simulink model "Check2_3"  (R2016b)
settings: Solver=VariableStepAuto  StartTime=0.0  StopTime=2  RelTol=1e-3
values from neighbouring files (symbols this model uses):
  h = 0.005    [Lab2.m]
  K = (K1 + K2) / 2    (= 15.4249961351)    [Lab2.m]
  kz1 = 15.2    [Lab2.m]
  kz2 = 4.22    [Lab2.m]
  kz3 = 1.73    [Lab2.m]
  tau = sqrt(tau1*tau2)    [Lab2.m]
  z1 = int(min_index)    [Lab2.m]
  z2 = z1 / 2    [Lab2.m]
  z3 = z1 / 3    [Lab2.m]
settings Model: Creator=EE103  LastModifiedBy=EE103

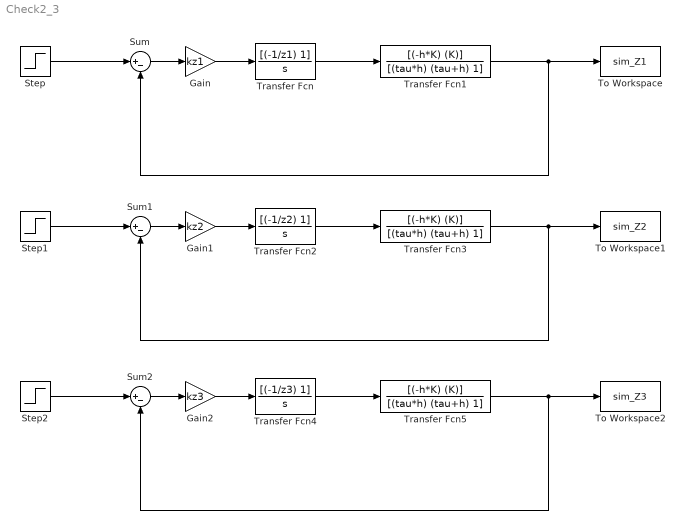
== system Check2_3 ==
  Gain : Gain  Gain=kz1
  Gain1 : Gain  Gain=kz2
  Gain2 : Gain  Gain=kz3
  Step : Step  Time=0  After=50  SampleTime=0.01
  Step1 : Step  Time=0  After=50  SampleTime=0.01
  Step2 : Step  Time=0  After=50  SampleTime=0.01
  Sum : Sum  Inputs=|+-
  Sum1 : Sum  Inputs=|+-
  Sum2 : Sum  Inputs=|+-
  To Workspace : ToWorkspace  VariableName=sim_Z1  SaveFormat=Timeseries  SampleTime=-1
  To Workspace1 : ToWorkspace  VariableName=sim_Z2  SaveFormat=Timeseries  SampleTime=-1
  To Workspace2 : ToWorkspace  VariableName=sim_Z3  SaveFormat=Timeseries  SampleTime=-1
  Transfer Fcn : TransferFcn  Numerator=[(-1/z1) 1]  Denominator=[1 0]
  Transfer Fcn1 : TransferFcn  Numerator=[(-h*K) (K)]  Denominator=[(tau*h) (tau+h) 1]
  Transfer Fcn2 : TransferFcn  Numerator=[(-1/z2) 1]  Denominator=[1 0]
  Transfer Fcn3 : TransferFcn  Numerator=[(-h*K) (K)]  Denominator=[(tau*h) (tau+h) 1]
  Transfer Fcn4 : TransferFcn  Numerator=[(-1/z3) 1]  Denominator=[1 0]
  Transfer Fcn5 : TransferFcn  Numerator=[(-h*K) (K)]  Denominator=[(tau*h) (tau+h) 1]
  wires:
  Step/1 -> Sum/1
  Sum/1 -> Gain/1
  Transfer Fcn/1 -> Transfer Fcn1/1
  Transfer Fcn1/1 -> Sum/2, To Workspace/1
  Step1/1 -> Sum1/1
  Sum1/1 -> Gain1/1
  Transfer Fcn2/1 -> Transfer Fcn3/1
  Transfer Fcn3/1 -> Sum1/2, To Workspace1/1
  Step2/1 -> Sum2/1
  Sum2/1 -> Gain2/1
  Transfer Fcn4/1 -> Transfer Fcn5/1
  Transfer Fcn5/1 -> Sum2/2, To Workspace2/1
  Gain/1 -> Transfer Fcn/1
  Gain1/1 -> Transfer Fcn2/1
  Gain2/1 -> Transfer Fcn4/1
